simulink model "Ex2_IC"  (R2021a)
settings: Solver=VariableStepAuto  StartTime=0.0  StopTime=10.0  RelTol=1e-3
libraries: dspfdesign x1
settings Model: Creator=gferr  LastModifiedBy=gferr

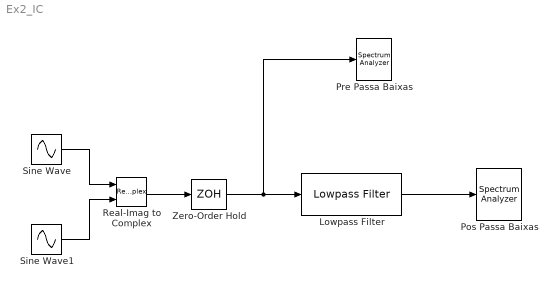
== system Ex2_IC ==
  Lowpass Filter : dspfdesign/Lowpass Filter  FilterType=FIR  DesignForMinimumOrder=on  FilterOrder=50  PassbandFrequency=3000  StopbandFrequency=8000  PassbandRipple=0.1  StopbandAttenuation=80  InheritSampleRate=off  SampleRate=100000  SimulateUsing=Interpreted execution  roundingMode=Floor  coeffsDataTypeStr=fixdt(1,16)
  Pos Passa Baixas : SpectrumAnalyzer
  Pre Passa Baixas : SpectrumAnalyzer
  Real-Imag to Complex : RealImagToComplex
  Sine Wave : Sin  Frequency=2*pi*1000  SampleTime=1e-4
  Sine Wave1 : Sin  TimeSource=Use external signal  Frequency=2*pi*1000  Phase=pi/2  SampleTime=1e-5
  Zero-Order Hold : ZeroOrderHold  SampleTime=1e-5
  wires:
  Zero-Order Hold/1 -> Pre Passa Baixas/1, Lowpass Filter/1
  Lowpass Filter/1 -> Pos Passa Baixas/1
  Sine Wave/1 -> Real-Imag to Complex/1
  Sine Wave1/1 -> Real-Imag to Complex/2
  Real-Imag to Complex/1 -> Zero-Order Hold/1
